simulink model "roll_loop"  (Simulink 7.4)
settings: Solver=ode45  StartTime=0.0  StopTime=30  RelTol=1e-3
values from neighbouring files (symbols this model uses):
  a_phi1 = den(2)    [computeGains.m]    (also in compute_tf_model.m = -0.5*rho*Va_trim^2*S_wing*b*C_p_p*b/2/Va_trim)
  a_phi2 = num(3)    [computeGains.m]    (also in compute_tf_model.m = 0.5*rho*Va_trim^2*S_wing*b*C_p_delta_a)
  delta_a_max = 45*pi/180    (= 0.785398163397)    [computeGains.m]
  P = varargin{5}    [my_mav_dynamics.m]
  phi_max = 15*pi/180    (= 0.261799387799)    [computeGains.m]
settings Model: Creator=beard  LastModifiedBy=beard

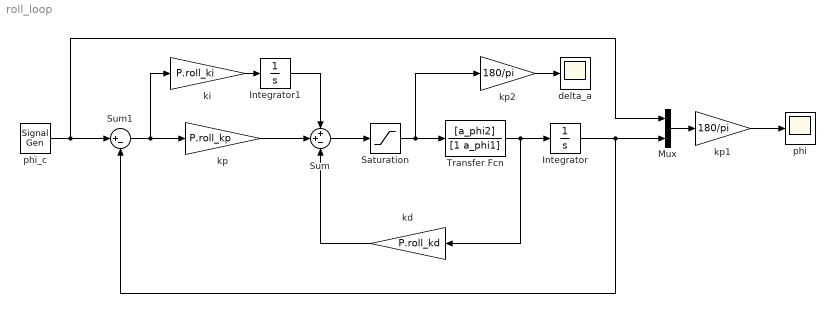
== system roll_loop ==
  Integrator : Integrator
  Integrator1 : Integrator
  Mux : Mux  Inputs=2
  Saturation : Saturate  UpperLimit=delta_a_max  LowerLimit=-delta_a_max  OutDataType=fixdt(1, 16)  OutScaling=2^0
  Sum : Sum  Inputs=++-  OutDataType=fixdt(1, 16)  OutScaling=2^0
  Sum1 : Sum  Inputs=|+-  OutDataType=fixdt(1, 16)  OutScaling=2^0
  Transfer Fcn : TransferFcn  Numerator=[a_phi2]  Denominator=[1 a_phi1]
  delta_a : Scope
      settings: TimeRange=30  YMin=-100  YMax=100
  kd : Gain  Gain=P.roll_kd  ParameterDataType=fixdt(1, 16)  ParameterScaling=2^0  OutDataType=fixdt(1, 16)  OutScaling=2^0
  ki : Gain  Gain=P.roll_ki  ParameterDataType=fixdt(1, 16)  ParameterScaling=2^0  OutDataType=fixdt(1, 16)  OutScaling=2^0
  kp : Gain  Gain=P.roll_kp  ParameterDataType=fixdt(1, 16)  ParameterScaling=2^0  OutDataType=fixdt(1, 16)  OutScaling=2^0
  kp1 : Gain  Gain=180/pi  ParameterDataType=fixdt(1, 16)  ParameterScaling=2^0  OutDataType=fixdt(1, 16)  OutScaling=2^0
  kp2 : Gain  Gain=180/pi  ParameterDataType=fixdt(1, 16)  ParameterScaling=2^0  OutDataType=fixdt(1, 16)  OutScaling=2^0
  phi : Scope
      settings: TimeRange=30  YMin=-40  YMax=40
  phi_c : SignalGenerator  WaveForm=square  Amplitude=phi_max  Frequency=.05
  wires:
  Transfer Fcn/1 -> Integrator/1, kd/1
  Saturation/1 -> Transfer Fcn/1, kp2/1
  Sum/1 -> Saturation/1
  kd/1 -> Sum/3
  kp/1 -> Sum/2
  Sum1/1 -> kp/1, ki/1
  ki/1 -> Integrator1/1
  Integrator1/1 -> Sum/1
  Integrator/1 -> Sum1/2, Mux/2
  phi_c/1 -> Sum1/1, Mux/1
  kp1/1 -> phi/1
  Mux/1 -> kp1/1
  kp2/1 -> delta_a/1
